simulink model "sim_1"  (R2020a)
settings: Solver=FixedStepAuto  StartTime=0.0  StopTime=10.0  FixedStep=0.05  RelTol=1e-3
values from neighbouring files (symbols this model uses):
  f_new = K*wi_lw    [computations.m]    (also in computations_better.m = gaussian_basis(s,1,500,50,f_s))
  y = sin(a*(t-3))    [computations.m]    (also in computations_better.m)
settings Model: Creator=sirius  LastModifiedBy=sirius

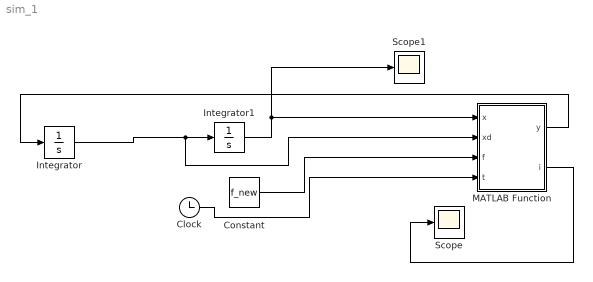
== system sim_1 ==
  Clock : Clock
  Constant : Constant  Value=f_new
  Integrator : Integrator
  Integrator1 : Integrator  InitialCondition=y(1)
  MATLAB Function : MATLAB Function  TreatAsAtomicUnit=on
  Scope : Scope
  Scope1 : Scope
  wires:
  Integrator/1 -> MATLAB Function/2(xd), Integrator1/1
  Integrator1/1 -> MATLAB Function/1(x), Scope1/1
  MATLAB Function/1(y) -> Integrator/1
  Constant/1 -> MATLAB Function/3(f)
  Clock/1 -> MATLAB Function/4(t)
  MATLAB Function/2(i) -> Scope/1

== matlab function sim_1/MATLAB Function ==
  data: x input; xd input; y output; f input; t input; i output
function [y,i]= fcn(x, xd, f, t)
i = round(t/0.05);

y = f(1+i);
